simulink model "ysw3_48"  (R2014a)
settings: Solver=ode45  StartTime=0.0  StopTime=10.0  RelTol=1e-3
settings Model: Creator=Administrator  LastModifiedBy=Administrator

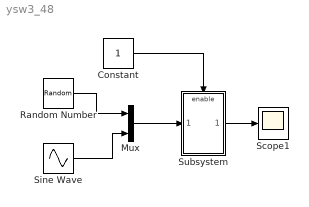
== system ysw3_48 ==
  Constant : Constant
  Mux : Mux  Inputs=2
  Random Number : RandomNumber  SampleTime=0.1
  Scope1 : Scope
      settings: TimeRange=10
  Sine Wave : Sin  SampleTime=0.1
  Subsystem : Subsystem
  wires:
  Random Number/1 -> Mux/1
  Sine Wave/1 -> Mux/2
  Mux/1 -> Subsystem/1(In1)
  Subsystem/1(Out1) -> Scope1/1
  Constant/1 -> Subsystem/Enable

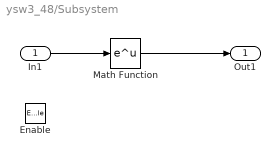
== system ysw3_48/Subsystem ==
  In1 : Inport
  Enable : EnablePort  StatesWhenEnabling=reset
  Math Function : Math  SaturateOnIntegerOverflow=on
  Out1 : Outport
  wires:
  Math Function/1 -> Out1/1
  In1/1 -> Math Function/1
